simulink model "ProjB_IntegratorModelB"  (R2024b)
settings: Solver=VariableStepAuto  StartTime=0.0  StopTime=10.0  RelTol=1e-3
settings Model: Creator=mlwu  LastModifiedBy=mlwu

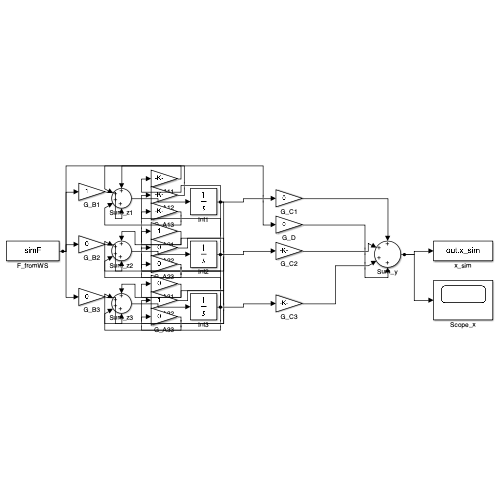
[thumbnail: Simulink's stored preview of the top-level diagram]
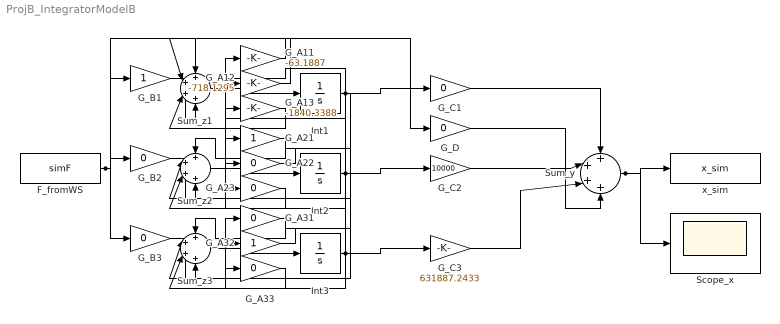
== system ProjB_IntegratorModelB ==
  F_fromWS : FromWorkspace  VariableName=simF
  G_A11 : Gain  Gain=-63.1887
  G_A12 : Gain  Gain=-718.1295
  G_A13 : Gain  Gain=-1840.3388
  G_A21 : Gain
  G_A{22..23,31,33} (4 alike) : Gain  Gain=0
  G_A32 : Gain
  G_B1 : Gain
  G_B2 : Gain  Gain=0
  G_B3 : Gain  Gain=0
  G_C1 : Gain  Gain=0
  G_C2 : Gain  Gain=10000
  G_C3 : Gain  Gain=631887.2433
  G_D : Gain  Gain=0
  Int1 : Integrator
  Int2 : Integrator
  Int3 : Integrator
  Scope_x : Scope
  Sum_y : Sum  Inputs=++++
  Sum_z1 : Sum  Inputs=++++
  Sum_z2 : Sum  Inputs=++++
  Sum_z3 : Sum  Inputs=++++
  x_sim : ToWorkspace  VariableName=x_sim  SaveFormat=Structure With Time  SampleTime=-1
  wires:
  Sum_z1/1 -> Int1/1
  Sum_z2/1 -> Int2/1
  Sum_z3/1 -> Int3/1
  Int1/1 -> G_A11/1, G_A21/1, G_A31/1, G_C1/1
  G_A11/1 -> Sum_z1/1
  Int2/1 -> G_A12/1, G_A22/1, G_A32/1, G_C2/1
  G_A12/1 -> Sum_z1/2
  Int3/1 -> G_A13/1, G_A23/1, G_A33/1, G_C3/1
  G_A13/1 -> Sum_z1/3
  F_fromWS/1 -> G_B1/1, G_B2/1, G_B3/1, G_D/1
  G_B1/1 -> Sum_z1/4
  G_A21/1 -> Sum_z2/1
  G_A22/1 -> Sum_z2/2
  G_A23/1 -> Sum_z2/3
  G_B2/1 -> Sum_z2/4
  G_A31/1 -> Sum_z3/1
  G_A32/1 -> Sum_z3/2
  G_A33/1 -> Sum_z3/3
  G_B3/1 -> Sum_z3/4
  G_C1/1 -> Sum_y/1
  G_C2/1 -> Sum_y/2
  G_C3/1 -> Sum_y/3
  G_D/1 -> Sum_y/4
  Sum_y/1 -> x_sim/1, Scope_x/1
